simulink model "EMI_Filter"  (R2024a)
settings: Solver=VariableStepAuto  StartTime=0.0  StopTime=0.1  RelTol=1e-3
libraries: spsSeriesRLCBranchLib x43, spsCurrentMeasurementLib x6, spsDiodeLib x3, spsDCVoltageSourceLib x3, spsMosfetLib x3, spsVoltageMeasurementLib x3, sps_lib x3, dspxfrm3 x1, eeGeneralControl x1, simulink x1, spsThreePhaseSeriesRLCBranchLib x1
settings Model: Creator=AEES-STUDENT  LastModifiedBy=AEES-STUDENT
settings SolverCC: ZeroCrossAlgorithm=Adaptive
settings DebuggingCC: IgnoredZcDiagnostic=none

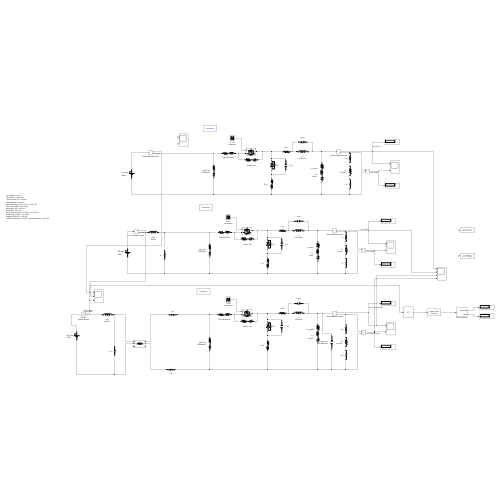
[thumbnail: Simulink's stored preview of the top-level diagram]
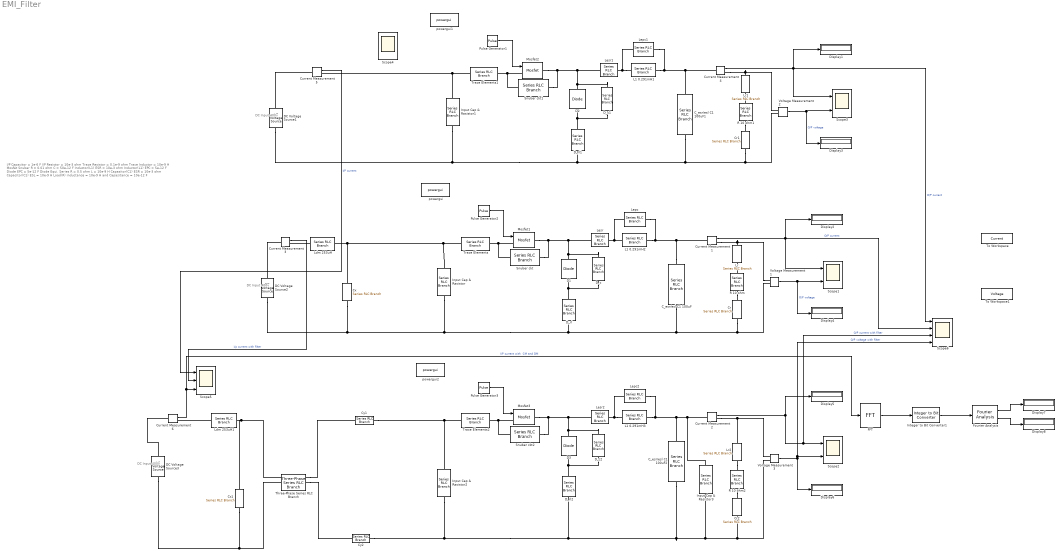
== system EMI_Filter ==
  note: I/P Capacitor = 1e-6 F
      | I/P Resistor = 10e-3 ohm
      | Trace Resistor = 0.1e-9 ohm
      | Trace Inductor = 10e-9 H
      | Mosfet Snuber R = 0.01 ohm  C = 50e-12 F
      | Inductor(L1) ESR = 10e-3 ohm
      | Inductor(L1) EPC = 5e-12 F
      | Diode EPC = 5e-12 F
      | Diode Equi. Series R = 0.5 ohm   L = 10e-9 H
      | Capasitor(C1) ESR = 10e-3 ohm
      | Capacitor(C1) ESL =  10e-9 H
      | Load(R) inductance = 10e-9 H   and Capasitance = 10e-12 F
  note: DC Input
      | 400v
  note: DC Input
      | 400v
  note: DC Input
      | 400v
  C_esr/esl C1 100uF : spsSeriesRLCBranchLib/Series RLC Branch  LConnTagsString=__new0  RConnTagsString=__new0  BranchType=RLC  Resistance=10e-3  Inductance=10e-9  SetiL0=off  InitialCurrent=0  Capacitance=100e-6  Setx0=off  InitialVoltage=0  Measurements=None
  C_esr/esl C1 100uF1 : spsSeriesRLCBranchLib/Series RLC Branch  LConnTagsString=__new0  RConnTagsString=__new0  BranchType=RLC  Resistance=10e-3  Inductance=10e-9  SetiL0=off  InitialCurrent=0  Capacitance=100e-6  Setx0=off  InitialVoltage=0  Measurements=None
  C_esr/esl C1 100uF2 : spsSeriesRLCBranchLib/Series RLC Branch  LConnTagsString=__new0  RConnTagsString=__new0  BranchType=RLC  Resistance=10e-3  Inductance=10e-9  SetiL0=off  InitialCurrent=0  Capacitance=100e-6  Setx0=off  InitialVoltage=0  Measurements=None
  Cr : spsSeriesRLCBranchLib/Series RLC Branch  LConnTagsString=__new0  RConnTagsString=__new0  BranchType=C  Resistance=10  Inductance=10e-9  SetiL0=off  InitialCurrent=0  Capacitance=10e-12  Setx0=off  InitialVoltage=0  Measurements=None
  Cr1 : spsSeriesRLCBranchLib/Series RLC Branch  LConnTagsString=__new0  RConnTagsString=__new0  BranchType=C  Resistance=10  Inductance=10e-9  SetiL0=off  InitialCurrent=0  Capacitance=10e-12  Setx0=off  InitialVoltage=0  Measurements=None
  Cr2 : spsSeriesRLCBranchLib/Series RLC Branch  LConnTagsString=__new0  RConnTagsString=__new0  BranchType=C  Resistance=10  Inductance=10e-9  SetiL0=off  InitialCurrent=0  Capacitance=10e-12  Setx0=off  InitialVoltage=0  Measurements=None
  Current Measurement{1..6} (6 alike) : spsCurrentMeasurementLib/Current Measurement  PhasorSimulation=off  OutputType=Complex  PSBequivalent=0
  Cx : spsSeriesRLCBranchLib/Series RLC Branch  LConnTagsString=__new0  RConnTagsString=__new0  BranchType=C  Resistance=10  Inductance=10e-9  SetiL0=off  InitialCurrent=0  Capacitance=1e-6  Setx0=off  InitialVoltage=0  Measurements=None
  Cx1 : spsSeriesRLCBranchLib/Series RLC Branch  LConnTagsString=__new0  RConnTagsString=__new0  BranchType=C  Resistance=10  Inductance=10e-9  SetiL0=off  InitialCurrent=0  Capacitance=1e-6  Setx0=off  InitialVoltage=0  Measurements=None
  Cy1 : spsSeriesRLCBranchLib/Series RLC Branch  LConnTagsString=__new0  RConnTagsString=__new0  BranchType=C  Resistance=10  Inductance=10e-9  SetiL0=off  InitialCurrent=0  Capacitance=2.2e-9  Setx0=off  InitialVoltage=0  Measurements=None
  Cy2 : spsSeriesRLCBranchLib/Series RLC Branch  LConnTagsString=__new0  RConnTagsString=__new0  BranchType=C  Resistance=10  Inductance=10e-9  SetiL0=off  InitialCurrent=0  Capacitance=2.2e-9  Setx0=off  InitialVoltage=0  Measurements=None
  D1 : spsDiodeLib/Diode  Ron=0.001  Lon=0  Vf=0.8  IC=0  UseSnubber=0  Rs=500  Cs=250e-9  Measurements=off
  D2 : spsDiodeLib/Diode  Ron=0.001  Lon=0  Vf=0.8  IC=0  UseSnubber=0  Rs=500  Cs=250e-9  Measurements=off
  D3 : spsDiodeLib/Diode  Ron=0.001  Lon=0  Vf=0.8  IC=0  UseSnubber=0  Rs=500  Cs=250e-9  Measurements=off
  DC Voltage Source1 : spsDCVoltageSourceLib/DC Voltage Source  Amplitude=400  Measurements=None
  DC Voltage Source2 : spsDCVoltageSourceLib/DC Voltage Source  Amplitude=400  Measurements=None
  DC Voltage Source3 : spsDCVoltageSourceLib/DC Voltage Source  Amplitude=400  Measurements=None
  D_c : spsSeriesRLCBranchLib/Series RLC Branch  LConnTagsString=__new0  RConnTagsString=__new0  BranchType=C  Resistance=0.1  Inductance=0.291e-3  SetiL0=off  InitialCurrent=0  Capacitance=5e-12  Setx0=off  InitialVoltage=0  Measurements=None
  D_c1 : spsSeriesRLCBranchLib/Series RLC Branch  LConnTagsString=__new0  RConnTagsString=__new0  BranchType=C  Resistance=0.1  Inductance=0.291e-3  SetiL0=off  InitialCurrent=0  Capacitance=5e-12  Setx0=off  InitialVoltage=0  Measurements=None
  D_c2 : spsSeriesRLCBranchLib/Series RLC Branch  LConnTagsString=__new0  RConnTagsString=__new0  BranchType=C  Resistance=0.1  Inductance=0.291e-3  SetiL0=off  InitialCurrent=0  Capacitance=5e-12  Setx0=off  InitialVoltage=0  Measurements=None
  D_rl : spsSeriesRLCBranchLib/Series RLC Branch  LConnTagsString=__new0  RConnTagsString=__new0  BranchType=RL  Resistance=0.5  Inductance=10e-9  SetiL0=off  InitialCurrent=0  Capacitance=100e-6  Setx0=off  InitialVoltage=0  Measurements=None
  D_rl1 : spsSeriesRLCBranchLib/Series RLC Branch  LConnTagsString=__new0  RConnTagsString=__new0  BranchType=RL  Resistance=0.5  Inductance=10e-9  SetiL0=off  InitialCurrent=0  Capacitance=100e-6  Setx0=off  InitialVoltage=0  Measurements=None
  D_rl2 : spsSeriesRLCBranchLib/Series RLC Branch  LConnTagsString=__new0  RConnTagsString=__new0  BranchType=RL  Resistance=0.5  Inductance=10e-9  SetiL0=off  InitialCurrent=0  Capacitance=100e-6  Setx0=off  InitialVoltage=0  Measurements=None
  Display{1..8} (8 alike) : Display
  FFT : dspxfrm3/FFT  FFTImplementation=Auto  CompMethod=Table lookup  TableOpt=NEW  TableOptActive=Speed  BitRevOrder=off  Normalize=off  InheritFFTLength=on  FFTLength=64  WrapInput=on  roundingMode=Ceiling  overflowMode=off  firstCoeffDataTypeStr=Inherit: Same word length as input  firstCoeffLastDataTypeStr=Inherit: Same word length as input  outputMin=[]  outputMax=[]
  Fourier Analysis : eeGeneralControl/Fourier Analysis  f=60  n=[1 2]  M0=1  Ph0=0  BufferSize=8192  Ts=-1
      settings: LibrarySourceBlock=ee_sl_lib/General Control/Fourier Analysis
  Input Cap & Rasistor : spsSeriesRLCBranchLib/Series RLC Branch  LConnTagsString=__new0  RConnTagsString=__new0  BranchType=RC  Resistance=10e-3  Inductance=0.1e-12  SetiL0=off  InitialCurrent=0  Capacitance=1e-6  Setx0=off  InitialVoltage=0  Measurements=None
  Input Cap & Rasistor1 : spsSeriesRLCBranchLib/Series RLC Branch  LConnTagsString=__new0  RConnTagsString=__new0  BranchType=RC  Resistance=10e-3  Inductance=0.1e-12  SetiL0=off  InitialCurrent=0  Capacitance=1e-6  Setx0=off  InitialVoltage=0  Measurements=None
  Input Cap & Rasistor2 : spsSeriesRLCBranchLib/Series RLC Branch  LConnTagsString=__new0  RConnTagsString=__new0  BranchType=RC  Resistance=10e-3  Inductance=0.1e-12  SetiL0=off  InitialCurrent=0  Capacitance=1e-6  Setx0=off  InitialVoltage=0  Measurements=None
  Input Cap & Rasistor3 : spsSeriesRLCBranchLib/Series RLC Branch  LConnTagsString=__new0  RConnTagsString=__new0  BranchType=C  Resistance=10e-3  Inductance=0.1e-12  SetiL0=off  InitialCurrent=0  Capacitance=1e-6  Setx0=off  InitialVoltage=0  Measurements=None
  Integer to Bit Converter1 : simulink/Logic and Bit Operations/Integer to Bit Converter  nbits=3  signedInputValues=Unsigned  bitOrder=MSB first  outDtype=Same as input
  L1 0.291mH1 : spsSeriesRLCBranchLib/Series RLC Branch  LConnTagsString=__new0  RConnTagsString=__new0  BranchType=L  Resistance=100e-3  Inductance=0.291e-3  SetiL0=off  InitialCurrent=0  Capacitance=1e-6  Setx0=off  InitialVoltage=0  Measurements=None
  L1 0.291mH2 : spsSeriesRLCBranchLib/Series RLC Branch  LConnTagsString=__new0  RConnTagsString=__new0  BranchType=L  Resistance=100e-3  Inductance=0.291e-3  SetiL0=off  InitialCurrent=0  Capacitance=1e-6  Setx0=off  InitialVoltage=0  Measurements=None
  L1 0.291mH3 : spsSeriesRLCBranchLib/Series RLC Branch  LConnTagsString=__new0  RConnTagsString=__new0  BranchType=L  Resistance=100e-3  Inductance=0.291e-3  SetiL0=off  InitialCurrent=0  Capacitance=1e-6  Setx0=off  InitialVoltage=0  Measurements=None
  Ldm 253uH : spsSeriesRLCBranchLib/Series RLC Branch  LConnTagsString=__new0  RConnTagsString=__new0  BranchType=L  Resistance=100e-3  Inductance=253e-6  SetiL0=off  InitialCurrent=0  Capacitance=1e-6  Setx0=off  InitialVoltage=0  Measurements=None
  Ldm 253uH1 : spsSeriesRLCBranchLib/Series RLC Branch  LConnTagsString=__new0  RConnTagsString=__new0  BranchType=L  Resistance=100e-3  Inductance=253e-6  SetiL0=off  InitialCurrent=0  Capacitance=1e-6  Setx0=off  InitialVoltage=0  Measurements=None
  Lepc : spsSeriesRLCBranchLib/Series RLC Branch  LConnTagsString=__new0  RConnTagsString=__new0  BranchType=C  Resistance=0.1  Inductance=0.291e-3  SetiL0=off  InitialCurrent=0  Capacitance=10e-12  Setx0=off  InitialVoltage=0  Measurements=None
  Lepc1 : spsSeriesRLCBranchLib/Series RLC Branch  LConnTagsString=__new0  RConnTagsString=__new0  BranchType=C  Resistance=0.1  Inductance=0.291e-3  SetiL0=off  InitialCurrent=0  Capacitance=10e-12  Setx0=off  InitialVoltage=0  Measurements=None
  Lepc2 : spsSeriesRLCBranchLib/Series RLC Branch  LConnTagsString=__new0  RConnTagsString=__new0  BranchType=C  Resistance=0.1  Inductance=0.291e-3  SetiL0=off  InitialCurrent=0  Capacitance=10e-12  Setx0=off  InitialVoltage=0  Measurements=None
  Lesr : spsSeriesRLCBranchLib/Series RLC Branch  LConnTagsString=__new0  RConnTagsString=__new0  BranchType=R  Resistance=10e-3  Inductance=1e-3  SetiL0=off  InitialCurrent=0  Capacitance=100e-6  Setx0=off  InitialVoltage=0  Measurements=None
  Lesr1 : spsSeriesRLCBranchLib/Series RLC Branch  LConnTagsString=__new0  RConnTagsString=__new0  BranchType=R  Resistance=10e-3  Inductance=1e-3  SetiL0=off  InitialCurrent=0  Capacitance=100e-6  Setx0=off  InitialVoltage=0  Measurements=None
  Lesr2 : spsSeriesRLCBranchLib/Series RLC Branch  LConnTagsString=__new0  RConnTagsString=__new0  BranchType=R  Resistance=10e-3  Inductance=1e-3  SetiL0=off  InitialCurrent=0  Capacitance=100e-6  Setx0=off  InitialVoltage=0  Measurements=None
  Lr : spsSeriesRLCBranchLib/Series RLC Branch  LConnTagsString=__new0  RConnTagsString=__new0  BranchType=L  Resistance=10  Inductance=10e-9  SetiL0=off  InitialCurrent=0  Capacitance=100e-6  Setx0=off  InitialVoltage=0  Measurements=None
  Lr1 : spsSeriesRLCBranchLib/Series RLC Branch  LConnTagsString=__new0  RConnTagsString=__new0  BranchType=L  Resistance=10  Inductance=10e-9  SetiL0=off  InitialCurrent=0  Capacitance=100e-6  Setx0=off  InitialVoltage=0  Measurements=None
  Lr2 : spsSeriesRLCBranchLib/Series RLC Branch  LConnTagsString=__new0  RConnTagsString=__new0  BranchType=L  Resistance=10  Inductance=10e-9  SetiL0=off  InitialCurrent=0  Capacitance=100e-6  Setx0=off  InitialVoltage=0  Measurements=None
  Mosfet1 : spsMosfetLib/Mosfet  Ron=0.03  Lon=0  Rd=0.03  Vfd=1.2  IC=0  Rs=9  Cs=1e-9  Measurements=off
  Mosfet2 : spsMosfetLib/Mosfet  Ron=0.03  Lon=0  Rd=0.03  Vfd=1.2  IC=0  Rs=9  Cs=1e-9  Measurements=off
  Mosfet3 : spsMosfetLib/Mosfet  Ron=0.03  Lon=0  Rd=0.03  Vfd=1.2  IC=0  Rs=9  Cs=1e-9  Measurements=off
  Pulse Generator1 : DiscretePulseGenerator  PulseType=Time based  Amplitude=15  Period=1/200000  PulseWidth=3.147
  Pulse Generator2 : DiscretePulseGenerator  PulseType=Time based  Amplitude=15  Period=1/200000  PulseWidth=3.147
  Pulse Generator3 : DiscretePulseGenerator  PulseType=Time based  Amplitude=15  Period=1/200000  PulseWidth=10
  R 10 ohm : spsSeriesRLCBranchLib/Series RLC Branch  LConnTagsString=__new0  RConnTagsString=__new0  BranchType=R  Resistance=10  Inductance=1e-3  SetiL0=off  InitialCurrent=0  Capacitance=100e-6  Setx0=off  InitialVoltage=0  Measurements=None
  R 10 ohm1 : spsSeriesRLCBranchLib/Series RLC Branch  LConnTagsString=__new0  RConnTagsString=__new0  BranchType=R  Resistance=10  Inductance=1e-3  SetiL0=off  InitialCurrent=0  Capacitance=100e-6  Setx0=off  InitialVoltage=0  Measurements=None
  R 10 ohm2 : spsSeriesRLCBranchLib/Series RLC Branch  LConnTagsString=__new0  RConnTagsString=__new0  BranchType=R  Resistance=10  Inductance=1e-3  SetiL0=off  InitialCurrent=0  Capacitance=100e-6  Setx0=off  InitialVoltage=0  Measurements=None
  Scope{1..4} (4 alike) : Scope  NumInputPorts=2
  Scope5 : Scope  NumInputPorts=3
  Scope6 : Scope  NumInputPorts=4
  Snuber ckt : spsSeriesRLCBranchLib/Series RLC Branch  LConnTagsString=__new0  RConnTagsString=__new0  BranchType=RC  Resistance=0.01  Inductance=0.291e-3  SetiL0=off  InitialCurrent=0  Capacitance=50e-12  Setx0=off  InitialVoltage=0  Measurements=None
  Snuber ckt1 : spsSeriesRLCBranchLib/Series RLC Branch  LConnTagsString=__new0  RConnTagsString=__new0  BranchType=RC  Resistance=0.01  Inductance=0.291e-3  SetiL0=off  InitialCurrent=0  Capacitance=50e-12  Setx0=off  InitialVoltage=0  Measurements=None
  Snuber ckt2 : spsSeriesRLCBranchLib/Series RLC Branch  LConnTagsString=__new0  RConnTagsString=__new0  BranchType=RC  Resistance=0.01  Inductance=0.291e-3  SetiL0=off  InitialCurrent=0  Capacitance=50e-12  Setx0=off  InitialVoltage=0  Measurements=None
  Three-Phase Series RLC Branch : spsThreePhaseSeriesRLCBranchLib/Three-Phase Series RLC Branch  LConnTagsString=A|B|C  RConnTagsString=A|B|C  BranchType=L  Resistance=1  Inductance=57.5e-3  Capacitance=1e-6  Measurements=None
  To Workspace : ToWorkspace  VariableName=Current  SaveFormat=Structure With Time  SampleTime=-1
  To Workspace1 : ToWorkspace  VariableName=Voltage  SaveFormat=Structure With Time  SampleTime=-1
  Trace Elements : spsSeriesRLCBranchLib/Series RLC Branch  LConnTagsString=__new0  RConnTagsString=__new0  BranchType=RL  Resistance=0.1e-9  Inductance=10e-9  SetiL0=off  InitialCurrent=0  Capacitance=100e-6  Setx0=off  InitialVoltage=0  Measurements=None
  Trace Elements1 : spsSeriesRLCBranchLib/Series RLC Branch  LConnTagsString=__new0  RConnTagsString=__new0  BranchType=RL  Resistance=0.1e-9  Inductance=10e-9  SetiL0=off  InitialCurrent=0  Capacitance=100e-6  Setx0=off  InitialVoltage=0  Measurements=None
  Trace Elements2 : spsSeriesRLCBranchLib/Series RLC Branch  LConnTagsString=__new0  RConnTagsString=__new0  BranchType=RL  Resistance=0.1e-9  Inductance=10e-9  SetiL0=off  InitialCurrent=0  Capacitance=100e-6  Setx0=off  InitialVoltage=0  Measurements=None
  Voltage Measurement1 : spsVoltageMeasurementLib/Voltage Measurement  PhasorSimulation=off  OutputType=Complex  PSBequivalent=0
  Voltage Measurement2 : spsVoltageMeasurementLib/Voltage Measurement  PhasorSimulation=off  OutputType=Complex  PSBequivalent=0
  Voltage Measurement3 : spsVoltageMeasurementLib/Voltage Measurement  PhasorSimulation=off  OutputType=Complex  PSBequivalent=0
  powergui : sps_lib/powergui  Priority=1  SimulationMode=Continuous  SampleTime=50e-6  frequency=60  Iterations=50  frequencyindice=0  Pbase=100e6  ErrMax=1e-4  UnitsV=kV  UnitsW=MW  buscounter=0  FunctionMessages=off  echomessages=off  EnableUseOfTLC=off  CurrentSourceSwitches=off  DisableSnubberDevices=off  DisableRonSwitches=off  DisableVfSwitches=off  DisplayEquations=off  AutomaticDiscreteSolvers=off  SolverType=Tustin/Backward Euler (TBE)  Interpol=off  ExternalGateDelay=off  methode=off  Ts=100  x0status=blocks  SPID=on  SwTol=0  HookPort=off  NonlinearTolerance=1e-4  nMaxIteration=100  ContinueOnMaxIteration=off  RestoreLinks=warning  ResistiveCurrentMeasurement=off  Frange=[0:2:500]  Ylog=off  Xlog=on  ShowGrid=off  save=off  variable=ZData  structure=0  ZoomFFT=off  StartTime=0.0  cycles=1  DisplayStyle=1  fundamental=60  FreqAxis=off  MaxFrequency=1000  frequencyindicesteady=1  RmsSteady=1  display=off
  powergui1 : sps_lib/powergui  Priority=1  SimulationMode=Continuous  SampleTime=50e-6  frequency=60  Iterations=50  frequencyindice=0  Pbase=100e6  ErrMax=1e-4  UnitsV=kV  UnitsW=MW  buscounter=0  FunctionMessages=off  echomessages=off  EnableUseOfTLC=off  CurrentSourceSwitches=off  DisableSnubberDevices=off  DisableRonSwitches=off  DisableVfSwitches=off  DisplayEquations=off  AutomaticDiscreteSolvers=off  SolverType=Tustin/Backward Euler (TBE)  Interpol=off  ExternalGateDelay=off  methode=off  Ts=100  x0status=blocks  SPID=on  SwTol=0  HookPort=off  NonlinearTolerance=1e-4  nMaxIteration=100  ContinueOnMaxIteration=off  RestoreLinks=warning  ResistiveCurrentMeasurement=off  Frange=[0:2:500]  Ylog=off  Xlog=on  ShowGrid=off  save=off  variable=ZData  structure=0  ZoomFFT=off  StartTime=0.0  cycles=1  DisplayStyle=1  fundamental=60  FreqAxis=off  MaxFrequency=1000  frequencyindicesteady=1  RmsSteady=1  display=off
  powergui2 : sps_lib/powergui  Priority=1  SimulationMode=Continuous  SampleTime=50e-6  frequency=60  Iterations=50  frequencyindice=0  Pbase=100e6  ErrMax=1e-4  UnitsV=kV  UnitsW=MW  buscounter=0  FunctionMessages=off  echomessages=off  EnableUseOfTLC=off  CurrentSourceSwitches=off  DisableSnubberDevices=off  DisableRonSwitches=off  DisableVfSwitches=off  DisplayEquations=off  AutomaticDiscreteSolvers=off  SolverType=Tustin/Backward Euler (TBE)  Interpol=off  ExternalGateDelay=off  methode=off  Ts=100  x0status=blocks  SPID=on  SwTol=0  HookPort=off  NonlinearTolerance=1e-4  nMaxIteration=100  ContinueOnMaxIteration=off  RestoreLinks=warning  ResistiveCurrentMeasurement=off  Frange=[0:2:500]  Ylog=off  Xlog=on  ShowGrid=off  save=off  variable=ZData  structure=0  ZoomFFT=off  StartTime=0.0  cycles=1  DisplayStyle=1  fundamental=60  FreqAxis=off  MaxFrequency=1000  frequencyindicesteady=1  RmsSteady=1  display=off
  wires:
  Pulse Generator2/1 -> Mosfet1/1
  Voltage Measurement1/1 -> Display4/1, Scope1/2  "O/P voltage"
  Current Measurement1/1 -> Scope1/1, Scope6/2, Display2/1  "O/P current"
  Current Measurement4/1 -> Scope3/1, Scope6/1, Display1/1  "O/P current"
  Pulse Generator1/1 -> Mosfet2/1
  Current Measurement5/1 -> Scope5/1  "I/P current"
  Voltage Measurement2/1 -> Scope3/2, Display3/1  "O/P voltage"
  Pulse Generator3/1 -> Mosfet3/1
  Current Measurement2/1 -> Scope6/3, Scope2/1, Display5/1  "O/P current with filter"
  Voltage Measurement3/1 -> Scope6/4, Scope2/2, Display6/1  "O/P voltage with filter"
  Current Measurement6/1 -> FFT/1, Scope5/3  "I/P current with  CM and DM"
  Current Measurement3/1 -> Scope5/2  "i/p current with filter"
  FFT/1 -> Integer to Bit Converter1/1
  Fourier Analysis/1 -> Display7/1
  Fourier Analysis/2 -> Display8/1
  Integer to Bit Converter1/1 -> Fourier Analysis/1
  connections:
  Voltage Measurement1/LConn2 -- Cr/RConn1 -- C_esr/esl C1 100uF/RConn1 -- Cx/RConn1 -- DC Voltage Source2/LConn1 -- Input Cap & Rasistor/RConn1 -- D_rl/RConn1
  C_esr/esl C1 100uF/LConn1 -- Current Measurement1/LConn1 -- Lepc/RConn1 -- L1 0.291mH2/RConn1
  D1/RConn1 -- Snuber ckt/RConn1 -- Mosfet1/RConn1 -- Lesr/LConn1 -- D_c/LConn1
  Voltage Measurement1/LConn1 -- Lr/LConn1 -- Current Measurement1/RConn1
  Mosfet1/LConn1 -- Snuber ckt/LConn1 -- Trace Elements/RConn1
  D_rl/LConn1 -- D_c/RConn1 -- D1/LConn1
  Ldm 253uH/LConn1 -- Current Measurement3/RConn1
  Lr/RConn1 -- R 10 ohm/LConn1
  R 10 ohm/RConn1 -- Cr/LConn1
  Lesr/RConn1 -- Lepc/LConn1 -- L1 0.291mH2/LConn1
  Trace Elements/LConn1 -- Cx/LConn1 -- Ldm 253uH/RConn1 -- Input Cap & Rasistor/LConn1
  Current Measurement3/LConn1 -- DC Voltage Source2/RConn1
  Trace Elements1/RConn1 -- Mosfet2/LConn1 -- Snuber ckt1/LConn1
  Input Cap & Rasistor1/LConn1 -- Trace Elements1/LConn1 -- Current Measurement5/RConn1
  L1 0.291mH1/LConn1 -- Lesr1/RConn1 -- Lepc1/LConn1
  Mosfet2/RConn1 -- D2/RConn1 -- D_c1/LConn1 -- Lesr1/LConn1 -- Snuber ckt1/RConn1
  D_rl1/RConn1 -- DC Voltage Source1/LConn1 -- Input Cap & Rasistor1/RConn1 -- C_esr/esl C1 100uF1/RConn1 -- Voltage Measurement2/LConn2 -- Cr1/RConn1
  Current Measurement4/RConn1 -- Voltage Measurement2/LConn1 -- Lr1/LConn1
  L1 0.291mH1/RConn1 -- C_esr/esl C1 100uF1/LConn1 -- Current Measurement4/LConn1 -- Lepc1/RConn1
  D2/LConn1 -- D_rl1/LConn1 -- D_c1/RConn1
  R 10 ohm1/RConn1 -- Cr1/LConn1
  Lr1/RConn1 -- R 10 ohm1/LConn1
  DC Voltage Source1/RConn1 -- Current Measurement5/LConn1
  Mosfet3/RConn1 -- Snuber ckt2/RConn1 -- Lesr2/LConn1 -- D3/RConn1 -- D_c2/LConn1
  L1 0.291mH3/LConn1 -- Lesr2/RConn1 -- Lepc2/LConn1
  Three-Phase Series RLC Branch/RConn2 -- Cy2/LConn1
  Trace Elements2/RConn1 -- Mosfet3/LConn1 -- Snuber ckt2/LConn1
  Current Measurement2/RConn1 -- Voltage Measurement3/LConn1 -- Lr2/LConn1
  L1 0.291mH3/RConn1 -- Lepc2/RConn1 -- Input Cap & Rasistor3/LConn1 -- Current Measurement2/LConn1 -- C_esr/esl C1 100uF2/LConn1
  D3/LConn1 -- D_rl2/LConn1 -- D_c2/RConn1
  R 10 ohm2/RConn1 -- Cr2/LConn1
  Lr2/RConn1 -- R 10 ohm2/LConn1
  DC Voltage Source3/RConn1 -- Current Measurement6/LConn1
  Input Cap & Rasistor2/LConn1 -- Cy1/LConn1 -- Trace Elements2/LConn1
  DC Voltage Source3/LConn1 -- Three-Phase Series RLC Branch/LConn2 -- Cx1/RConn1
  Three-Phase Series RLC Branch/LConn1 -- Cx1/LConn1 -- Ldm 253uH1/RConn1
  Ldm 253uH1/LConn1 -- Current Measurement6/RConn1
  Three-Phase Series RLC Branch/RConn1 -- Cy1/RConn1
  C_esr/esl C1 100uF2/RConn1 -- Voltage Measurement3/LConn2 -- Cr2/RConn1 -- Input Cap & Rasistor3/RConn1 -- Cy2/RConn1 -- Input Cap & Rasistor2/RConn1 -- D_rl2/RConn1
